simulink model "Misil_Simulink"  (R2021b)
settings: Solver=ode45  StartTime=0.0  StopTime=10  RelTol=1e-3  EnableMultiTasking=on
PreLoadFcn:
  | codigos
undefined symbols (not defined in the file): b_ala, b_est, c, Cd0, CL0, Cl_deltaa, Cl_p, CLalpha, Cm_deltae, Cm_fq, Cm_w, Cn_deltar, Cn_fr, Cn_v, e, g, h, Ix, Ixz, Iy, Iz, L_ala, L_est, Long, m
libraries: aerolibanim x1, aerolibatmos2 x1
settings Model: Creator=usuario  LastModifiedBy=verti
settings SolverCC: AlgebraicLoopSolver=TrustRegion
settings DataIOCC: LimitDataPoints=on  SaveFormat=Array  SignalLoggingSaveFormat=ModelDataLogs  ReturnWorkspaceOutputs=off
settings OptimizationCC: ExpressionDepthLimit=2147483647  LifeSpan=inf
settings DebuggingCC: UnderspecifiedInitializationDetection=Classic  MergeDetectMultiDrivingBlocksExec=none  SolverPrmCheckMsg=warning  FcnCallInpInsideContextMsg=warning  StateNameClashWarn=warning  SFUnexpectedBacktrackingDiag=warning  SFNoUnconditionalDefaultTransitionDiag=warning  SFExecutionAtInitializationDiag=none  SFMachineParentedDataDiag=warning  ArithmeticOperatorsInVariantConditions=warning
settings HardwareCC: ProdBitPerPointer=32  ProdBitPerSizeT=32  ProdBitPerPtrDiffT=32  ProdLargestAtomicFloat=None  ProdIntDivRoundTo=Undefined  ProdEndianess=Unspecified  ProdWordSize=32  ProdHWDeviceType=32-bit Generic
settings ModelReferenceCC: PropagateSignalLabelsOutOfModel=off
settings SFSimCC: SimUseLocalCustomCode=off  CustomCodeUndefinedFunction=UseInterfaceOnly
settings RTWCC: RTWUseLocalCustomCode=off
settings CodeAppCC: StateflowObjectComments=on
settings GRTTargetCC: TargetLangStandard=C89/C90 (ANSI)  CombineOutputUpdateFcns=off  GRTInterface=on
settings ConfigComp: CovMetricSettings=dw  CovSaveCumulativeToWorkspaceVar=on  CovSaveSingleToWorkspaceVar=on  CovExternalEMLEnable=off

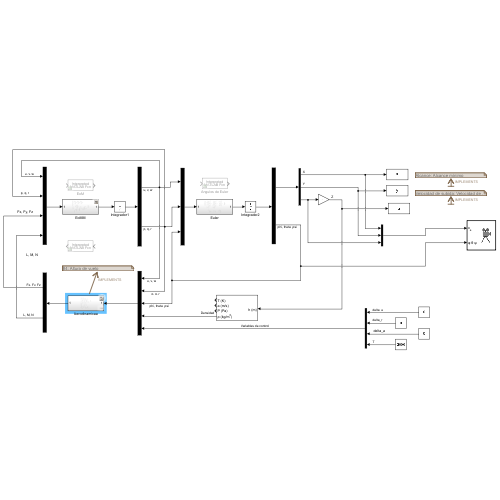
[thumbnail: Simulink's stored preview of the top-level diagram]
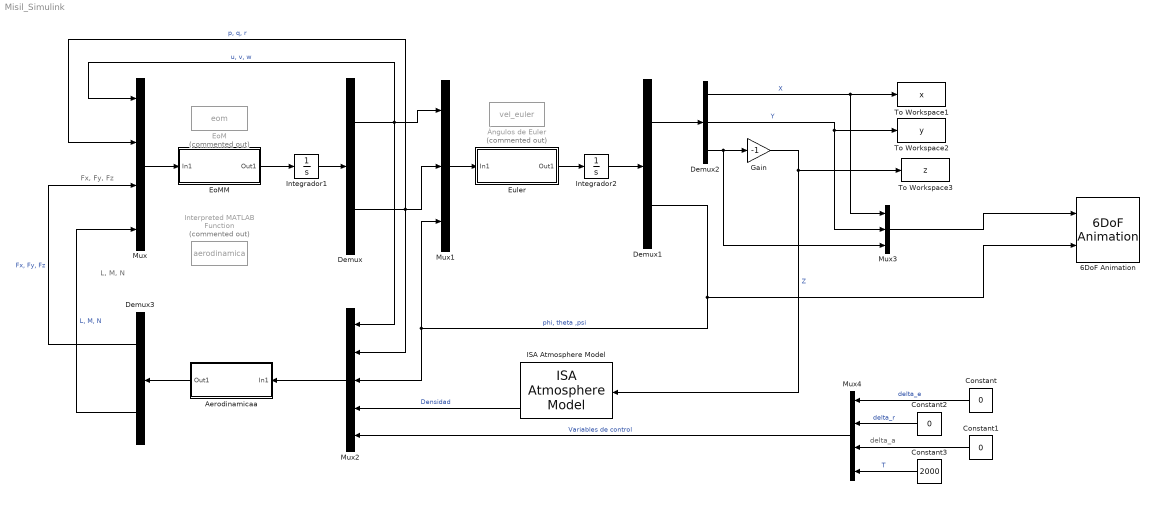
== system Misil_Simulink ==
  note: delta_a
  note: Fx, Fy, Fz
  note: L, M, N
  6DoF Animation : aerolibanim/6DoF Animation  u1=[0 4000 0 4000 0 4000]  u2=0.1  u3=20  u4=[0 0 0]  u5=Fly alongside  u6=[200 200 200]  u7=10  u8=on
  Aerodinamicaa : Subsystem
  Constant : Constant  Value=0
  Constant1 : Constant  Value=0
  Constant2 : Constant  Value=0
  Constant3 : Constant  Value=2000
  Demux : Demux  Outputs=2
  Demux1 : Demux  Outputs=2
  Demux2 : Demux  Outputs=3
  Demux3 : Demux  Outputs=2
  EoM : MATLABFcn  Commented=on  MATLABFcn=eom  OutputDimensions=6
  EoMM : Subsystem
  Euler : Subsystem
  Gain : Gain  Gain=-1
  ISA Atmosphere Model : aerolibatmos2/ISA Atmosphere Model  custom=off  g=9.80665  gamma=1.4  R=287.0531  L=0.0065  h_trop=11000  h_strat=20000  rho0=1.225  P0=101325  T0=288.15  h0=0
  Integrador1 : Integrator  InitialCondition=[0.001,0,0,0,0,0]
  Integrador2 : Integrator  InitialCondition=[0,0,2000,0,pi/4,0]
      settings: DeleteFcn=slcm Cancel;  NameChangeFcn=slcm Rename;
  Interpreted MATLAB Function : MATLABFcn  Commented=on  MATLABFcn=aerodinamica  OutputDimensions=6
  Mux : Mux
  Mux1 : Mux  Inputs=3
  Mux2 : Mux  Inputs=5
  Mux3 : Mux  Inputs=3
  Mux4 : Mux
  To Workspace1 : ToWorkspace  VariableName=x  SampleTime=-1
  To Workspace2 : ToWorkspace  VariableName=y  SampleTime=-1
  To Workspace3 : ToWorkspace  VariableName=z  SampleTime=-1
  Ángulos de Euler : MATLABFcn  Commented=on  MATLABFcn=vel_euler  OutputDimensions=6
  wires:
  Integrador1/1 -> Demux/1
  Mux1/1 -> Euler/1(In1)
  Integrador2/1 -> Demux1/1
  Demux1/1 -> Demux2/1
  Demux/2 -> Mux2/2, Mux/2, Mux1/2  "p, q, r"
  Demux1/2 -> 6DoF Animation/2, Mux2/3, Mux1/3  "phi, theta ,psi"
  Demux2/3 -> Gain/1, Mux3/3
  Gain/1 -> ISA Atmosphere Model/1, To Workspace3/1  "Z"
  Demux2/1 -> Mux3/1, To Workspace1/1  "X"
  Demux2/2 -> Mux3/2, To Workspace2/1  "Y"
  Constant3/1 -> Mux4/4  "T"
  Constant1/1 -> Mux4/3
  Constant2/1 -> Mux4/2  "delta_r"
  Constant/1 -> Mux4/1  "delta_e"
  Demux3/1 -> Mux/3  "Fx, Fy, Fz"
  Demux3/2 -> Mux/4  "L, M, N"
  ISA Atmosphere Model/4 -> Mux2/4  "Densidad"
  Mux4/1 -> Mux2/5  "Variables de control"
  Mux3/1 -> 6DoF Animation/1
  Demux/1 -> Mux2/1, Mux/1, Mux1/1  "u, v, w"
  Mux2/1 -> Aerodinamicaa/1(In1)
  Aerodinamicaa/1(Out1) -> Demux3/1
  Mux/1 -> EoMM/1(In1)
  EoMM/1(Out1) -> Integrador1/1
  Euler/1(Out1) -> Integrador2/1

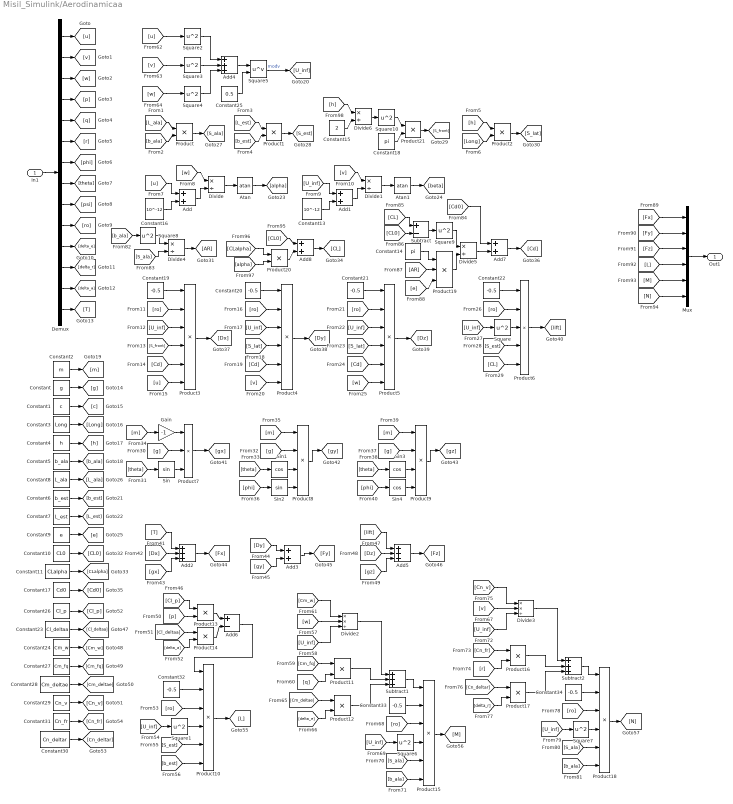
== system Misil_Simulink/Aerodinamicaa ==
  In1 : Inport
  Add{,1,3,7..8} (5 alike) : Sum
  Add2 : Sum  Inputs=+++
  Add4 : Sum  Inputs=+++
  Add5 : Sum  Inputs=+++
  Add6 : Sum  Inputs=+-
  Atan : Trigonometry  Operator=atan
  Atan1 : Trigonometry  Operator=atan
  Constant : Constant  Value=g
  Constant1 : Constant  Value=c
  Constant10 : Constant  Value=CL0
  Constant11 : Constant  Value=CLalpha
  Constant13 : Constant  Value=10^-12
  Constant14 : Constant  Value=pi
  Constant15 : Constant  Value=2
  Constant16 : Constant  Value=10^-12
  Constant17 : Constant  Value=Cd0
  Constant18 : Constant  Value=pi
  Constant{19..22,32..34} (7 alike) : Constant  Value=-0.5
  Constant2 : Constant  Value=m
  Constant23 : Constant  Value=Cl_deltaa
  Constant24 : Constant  Value=Cm_w
  Constant25 : Constant  Value=0.5
  Constant26 : Constant  Value=Cl_p
  Constant27 : Constant  Value=Cm_fq
  Constant28 : Constant  Value=Cm_deltae
  Constant29 : Constant  Value=Cn_v
  Constant3 : Constant  Value=Long
  Constant30 : Constant  Value=Cn_deltar
  Constant31 : Constant  Value=Cn_fr
  Constant4 : Constant  Value=h
  Constant5 : Constant  Value=b_ala
  Constant6 : Constant  Value=b_est
  Constant7 : Constant  Value=L_est
  Constant8 : Constant  Value=L_ala
  Constant9 : Constant  Value=e
  Demux : Demux  Outputs=14
  Divide{,1,4..6} (5 alike) : Product  Inputs=*/
  Divide2 : Product  Inputs=**/
  Divide3 : Product  Inputs=**/
  Gain : Gain  Gain=-1
  Mux : Mux  Inputs=6
  Product{,1..2,11..14,16..17,20..21} (11 alike) : Product
  Product{3..5,10,15,18} (6 alike) : Product  Inputs=6
  Product19 : Product  Inputs=3
  Product6 : Product  Inputs=5
  Product7 : Product  Inputs=3
  Product8 : Product  Inputs=4
  Product9 : Product  Inputs=4
  Sin : Trigonometry
  Sin1 : Trigonometry  Operator=cos
  Sin2 : Trigonometry
  Sin3 : Trigonometry  Operator=cos
  Sin4 : Trigonometry  Operator=cos
  Square{,1..4,6..10} (10 alike) : Math  Operator=square  SaturateOnIntegerOverflow=on
  Square5 : Math  Operator=pow  SaturateOnIntegerOverflow=on
  Subtract : Sum  Inputs=+-
  Subtract1 : Sum  Inputs=+++
  Subtract2 : Sum  Inputs=+++
  Out1 : Outport
  wires:
  In1/1 -> Demux/1
  Mux/1 -> Out1/1
  Demux/1 -> [u]
  Demux/2 -> [v]
  Demux/6 -> [r]
  Demux/5 -> [q]
  Demux/4 -> [p]
  Demux/3 -> [w]
  Demux/7 -> [phi]
  Demux/14 -> [T]
  Demux/13 -> [delta_a]
  Demux/12 -> [delta_r]
  Demux/11 -> [delta_e]
  Demux/10 -> [ro]
  Demux/9 -> [psi]
  Demux/8 -> [theta]
  Constant3/1 -> [Long]
  Constant2/1 -> [m]
  Constant/1 -> [g]
  Constant4/1 -> [h]
  Constant5/1 -> [b_ala]
  Constant1/1 -> [c]
  Add4/1 -> Square5/1
  Square5/1 -> [U_inf]  "modv"
  Constant25/1 -> Square5/2
  Square3/1 -> Add4/2
  [w] -> Square4/1
  [v] -> Square3/1
  Square4/1 -> Add4/3
  Square2/1 -> Add4/1
  [u] -> Square2/1
  Constant7/1 -> [L_est]
  Constant11/1 -> [CLalpha]
  Constant10/1 -> [CL0]
  Constant6/1 -> [b_est]
  Constant9/1 -> [e]
  [L_ala] -> Product/1
  [b_ala] -> Product/2
  Product/1 -> [S_ala]
  Product1/1 -> [S_est]
  [b_est] -> Product1/2
  [L_est] -> Product1/1
  [h] -> Product2/1
  Product2/1 -> [S_lat]
  [Long] -> Product2/2
  [u] -> Add/1
  Divide/1 -> Atan/1
  Add/1 -> Divide/2
  Atan/1 -> [alpha]
  [w] -> Divide/1
  Constant16/1 -> Add/2
  Constant13/1 -> Add1/2
  [v] -> Divide1/1
  Atan1/1 -> [beta]
  Add1/1 -> Divide1/2
  Divide1/1 -> Atan1/1
  [U_inf] -> Add1/1
  Divide4/1 -> [AR]
  Constant17/1 -> [Cd0]
  [U_inf] -> Product3/3
  [ro] -> Product3/2
  [Cd] -> Product3/5
  Constant19/1 -> Product3/1
  Product3/1 -> [Dx]
  [u] -> Product3/6
  [S_front] -> Product3/4
  [S_lat] -> Product4/4
  [v] -> Product4/6
  Product4/1 -> [Dy]
  Constant20/1 -> Product4/1
  [Cd] -> Product4/5
  [ro] -> Product4/2
  [U_inf] -> Product4/3
  [U_inf] -> Product5/3
  [ro] -> Product5/2
  [Cd] -> Product5/5
  Constant21/1 -> Product5/1
  Product5/1 -> [Dz]
  [w] -> Product5/6
  [S_lat] -> Product5/4
  [S_est] -> Product6/4
  Product6/1 -> [lift]
  Constant22/1 -> Product6/1
  [CL] -> Product6/5
  [ro] -> Product6/2
  [U_inf] -> Square/1
  Square/1 -> Product6/3
  Gain/1 -> Product7/1
  [g] -> Product7/2
  [theta] -> Sin/1
  Sin/1 -> Product7/3
  Product7/1 -> [gx]
  Product8/1 -> [gy]
  Sin1/1 -> Product8/3
  [theta] -> Sin1/1
  [g] -> Product8/2
  [m] -> Product8/1
  [m] -> Gain/1
  [phi] -> Sin2/1
  Sin2/1 -> Product8/4
  Sin4/1 -> Product9/4
  [phi] -> Sin4/1
  [m] -> Product9/1
  [g] -> Product9/2
  [theta] -> Sin3/1
  Sin3/1 -> Product9/3
  Product9/1 -> [gz]
  [T] -> Add2/1
  [Dx] -> Add2/2
  [gx] -> Add2/3
  Add2/1 -> [Fx]
  [gy] -> Add3/2
  Add3/1 -> [Fy]
  [Dy] -> Add3/1
  [lift] -> Add5/1
  Add5/1 -> [Fz]
  [gz] -> Add5/3
  [Dz] -> Add5/2
  Constant30/1 -> [Cn_deltar]
  Constant24/1 -> [Cm_w]
  Constant29/1 -> [Cn_v]
  Constant28/1 -> [Cm_deltae]
  Constant23/1 -> [Cl_deltaa]
  Constant26/1 -> [Cl_p]
  Constant27/1 -> [Cm_fq]
  Constant31/1 -> [Cn_fr]
  [Cl_p] -> Product13/1
  Product14/1 -> Add6/2
  [Cl_deltaa] -> Product14/1
  [p] -> Product13/2
  [delta_a] -> Product14/2
  [ro] -> Product10/3
  Square1/1 -> Product10/4
  [b_est] -> Product10/6
  Constant32/1 -> Product10/2
  Add6/1 -> Product10/1
  [U_inf] -> Square1/1
  Product10/1 -> [L]
  Product13/1 -> Add6/1
  [S_est] -> Product10/5
  Product15/1 -> [M]
  [Cm_fq] -> Product11/1
  [Cm_w] -> Divide2/1
  [S_ala] -> Product15/5
  [U_inf] -> Square6/1
  Divide2/1 -> Subtract1/1
  [w] -> Divide2/2
  [b_ala] -> Product15/6
  [ro] -> Product15/3
  Subtract1/1 -> Product15/1
  [U_inf] -> Divide2/3
  Constant33/1 -> Product15/2
  Product11/1 -> Subtract1/2
  [q] -> Product11/2
  Square6/1 -> Product15/4
  [delta_e] -> Product12/2
  [Cm_deltae] -> Product12/1
  Product12/1 -> Subtract1/3
  Product17/1 -> Subtract2/3
  [Cn_deltar] -> Product17/1
  [delta_r] -> Product17/2
  Square7/1 -> Product18/4
  [r] -> Product16/2
  Product16/1 -> Subtract2/2
  Constant34/1 -> Product18/2
  [U_inf] -> Divide3/3
  Subtract2/1 -> Product18/1
  [ro] -> Product18/3
  [b_ala] -> Product18/6
  [v] -> Divide3/2
  Divide3/1 -> Subtract2/1
  [U_inf] -> Square7/1
  [S_ala] -> Product18/5
  [Cn_v] -> Divide3/1
  [Cn_fr] -> Product16/1
  Product18/1 -> [N]
  [b_ala] -> Square8/1
  [S_ala] -> Divide4/2
  Square8/1 -> Divide4/1
  Add7/1 -> [Cd]
  [Cd0] -> Add7/1
  [CL0] -> Subtract/2
  [CL] -> Subtract/1
  Subtract/1 -> Square9/1
  Square9/1 -> Divide5/1
  Product19/1 -> Divide5/2
  Constant14/1 -> Product19/1
  [AR] -> Product19/2
  [e] -> Product19/3
  Divide5/1 -> Add7/2
  [Fx] -> Mux/1
  [Fy] -> Mux/2
  [Fz] -> Mux/3
  [L] -> Mux/4
  [M] -> Mux/5
  [N] -> Mux/6
  Add8/1 -> [CL]
  Product20/1 -> Add8/2
  [CL0] -> Add8/1
  [alpha] -> Product20/2
  [CLalpha] -> Product20/1
  [h] -> Divide6/1
  Constant15/1 -> Divide6/2
  Product21/1 -> [S_front]
  Divide6/1 -> Square10/1
  Constant18/1 -> Product21/2
  Square10/1 -> Product21/1
  Constant8/1 -> [L_ala]

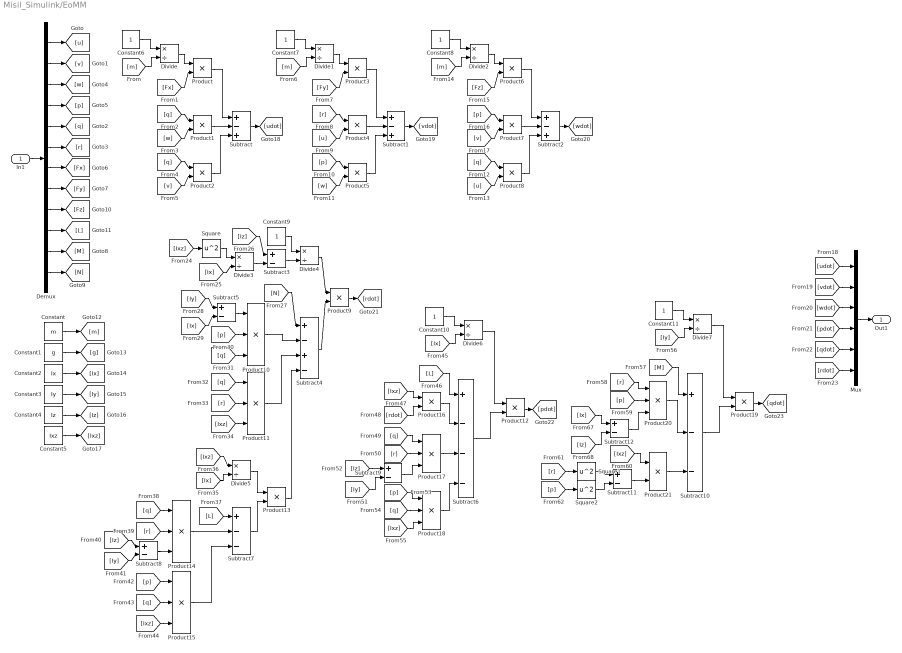
== system Misil_Simulink/EoMM ==
  In1 : Inport
  Constant : Constant  Value=m
  Constant1 : Constant  Value=g
  Constant{6..11} (6 alike) : Constant
  Constant2 : Constant  Value=Ix
  Constant3 : Constant  Value=Iy
  Constant4 : Constant  Value=Iz
  Constant5 : Constant  Value=Ixz
  Demux : Demux  Outputs=12
  Divide{,1..7} (8 alike) : Product  Inputs=*/
  Mux : Mux  Inputs=6
  Product{,1..9,12..13,16,19,21} (15 alike) : Product
  Product{10..11,14..15,17..18,20} (7 alike) : Product  Inputs=3
  Square : Math  Operator=square  SaturateOnIntegerOverflow=on
  Square1 : Math  Operator=square  SaturateOnIntegerOverflow=on
  Square2 : Math  Operator=square  SaturateOnIntegerOverflow=on
  Subtract : Sum  Inputs=+-+
  Subtract1 : Sum  Inputs=+-+
  Subtract10 : Sum  Inputs=+--
  Subtract{3,5,8..9,11..12} (6 alike) : Sum  Inputs=+-
  Subtract2 : Sum  Inputs=+-+
  Subtract4 : Sum  Inputs=+-+-
  Subtract6 : Sum  Inputs=+---
  Subtract7 : Sum  Inputs=+--
  Out1 : Outport
  wires:
  In1/1 -> Demux/1
  Demux/3 -> [w]
  Demux/1 -> [u]
  Demux/2 -> [v]
  Demux/4 -> [p]
  Demux/5 -> [q]
  Demux/6 -> [r]
  Demux/7 -> [Fx]
  Demux/12 -> [N]
  Demux/11 -> [M]
  Demux/10 -> [L]
  Demux/9 -> [Fz]
  Demux/8 -> [Fy]
  Constant/1 -> [m]
  Constant1/1 -> [g]
  Constant3/1 -> [Iy]
  Constant2/1 -> [Ix]
  Constant5/1 -> [Ixz]
  Constant4/1 -> [Iz]
  Constant6/1 -> Divide/1
  [m] -> Divide/2
  [Fx] -> Product/2
  Divide/1 -> Product/1
  [q] -> Product1/1
  [w] -> Product1/2
  [q] -> Product2/1
  [v] -> Product2/2
  Product2/1 -> Subtract/3
  Product/1 -> Subtract/1
  Product1/1 -> Subtract/2
  Subtract/1 -> [udot]
  Subtract1/1 -> [vdot]
  Product4/1 -> Subtract1/2
  Product3/1 -> Subtract1/1
  Product5/1 -> Subtract1/3
  [w] -> Product5/2
  [p] -> Product5/1
  [u] -> Product4/2
  [r] -> Product4/1
  Divide1/1 -> Product3/1
  [Fy] -> Product3/2
  [m] -> Divide1/2
  Constant7/1 -> Divide1/1
  Constant8/1 -> Divide2/1
  [m] -> Divide2/2
  [Fz] -> Product6/2
  Divide2/1 -> Product6/1
  [p] -> Product7/1
  [v] -> Product7/2
  [q] -> Product8/1
  [u] -> Product8/2
  Product8/1 -> Subtract2/3
  Product6/1 -> Subtract2/1
  Product7/1 -> Subtract2/2
  Subtract2/1 -> [wdot]
  [rdot] -> Mux/6
  Mux/1 -> Out1/1
  [udot] -> Mux/1
  [vdot] -> Mux/2
  [wdot] -> Mux/3
  [pdot] -> Mux/4
  [qdot] -> Mux/5
  [Ixz] -> Square/1
  Square/1 -> Divide3/1
  [Ix] -> Divide3/2
  [Iz] -> Subtract3/1
  Divide3/1 -> Subtract3/2
  Subtract3/1 -> Divide4/2
  Constant9/1 -> Divide4/1
  Divide4/1 -> Product9/1
  Subtract4/1 -> Product9/2
  [N] -> Subtract4/1
  [Iy] -> Subtract5/1
  [Ix] -> Subtract5/2
  Subtract5/1 -> Product10/1
  Product10/1 -> Subtract4/2
  [p] -> Product10/2
  [q] -> Product10/3
  [Ixz] -> Product11/3
  [r] -> Product11/2
  Product11/1 -> Subtract4/3
  [q] -> Product11/1
  [Ix] -> Divide5/2
  [Ixz] -> Divide5/1
  Product13/1 -> Subtract4/4
  Divide5/1 -> Product13/1
  Subtract7/1 -> Product13/2
  [L] -> Subtract7/1
  Product14/1 -> Subtract7/2
  Subtract8/1 -> Product14/3
  [q] -> Product14/1
  [r] -> Product14/2
  [Iz] -> Subtract8/1
  [Iy] -> Subtract8/2
  [q] -> Product15/2
  [p] -> Product15/1
  Product15/1 -> Subtract7/3
  [Ixz] -> Product15/3
  Product9/1 -> [rdot]
  Product12/1 -> [pdot]
  [Ix] -> Divide6/2
  Constant10/1 -> Divide6/1
  Divide6/1 -> Product12/1
  Subtract6/1 -> Product12/2
  [L] -> Subtract6/1
  [Ixz] -> Product16/1
  [rdot] -> Product16/2
  Product16/1 -> Subtract6/2
  Product17/1 -> Subtract6/3
  [q] -> Product17/1
  [r] -> Product17/2
  Subtract9/1 -> Product17/3
  [Iz] -> Subtract9/1
  [Iy] -> Subtract9/2
  [q] -> Product18/2
  [p] -> Product18/1
  [Ixz] -> Product18/3
  Product18/1 -> Subtract6/4
  [Ixz] -> Product21/1
  Product21/1 -> Subtract10/3
  Product20/1 -> Subtract10/2
  [M] -> Subtract10/1
  Subtract10/1 -> Product19/2
  Divide7/1 -> Product19/1
  Constant11/1 -> Divide7/1
  [Iy] -> Divide7/2
  Product19/1 -> [qdot]
  [r] -> Product20/1
  [p] -> Product20/2
  Subtract12/1 -> Product20/3
  [Ix] -> Subtract12/1
  [Iz] -> Subtract12/2
  Subtract11/1 -> Product21/2
  [r] -> Square1/1
  [p] -> Square2/1
  Square2/1 -> Subtract11/2
  Square1/1 -> Subtract11/1

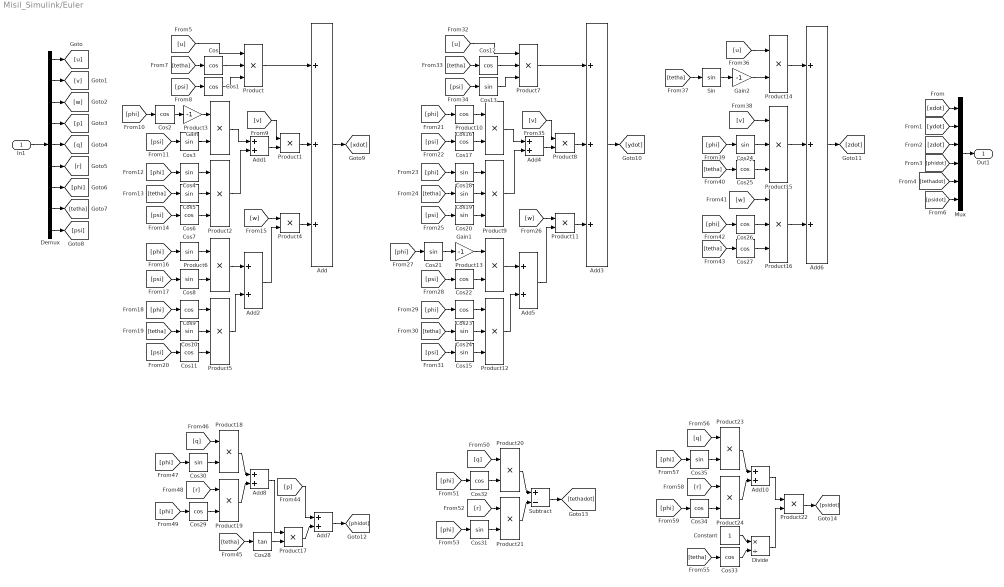
== system Misil_Simulink/Euler ==
  In1 : Inport
  Add : Sum  Inputs=+++
  Add{1..2,4..5,7..8,10} (7 alike) : Sum
  Add3 : Sum  Inputs=+++
  Add6 : Sum  Inputs=+++
  Constant : Constant
  Cos{,1..2,6,9,11..12,16..17,22..23,25..27,29,32..34} (18 alike) : Trigonometry  Operator=cos
  Cos{3..5,7..8,10,13..15,18..21,24,30..31,35} (17 alike) : Trigonometry
  Cos28 : Trigonometry  Operator=tan
  Demux : Demux  Outputs=9
  Divide : Product  Inputs=*/
  Gain : Gain  Gain=-1
  Gain1 : Gain  Gain=-1
  Gain2 : Gain  Gain=-1
  Mux : Mux  Inputs=6
  Product{,2,5,7,9,12,15..16} (8 alike) : Product  Inputs=3
  Product{1,3..4,6,8,10..11,13..14,17..24} (17 alike) : Product
  Sin : Trigonometry
  Subtract : Sum  Inputs=+-
  Out1 : Outport
  wires:
  In1/1 -> Demux/1
  Demux/1 -> [u]
  Demux/2 -> [v]
  Demux/3 -> [w]
  Demux/4 -> [p]
  Demux/5 -> [q]
  Demux/6 -> [r]
  Demux/7 -> [phi]
  Demux/8 -> [tetha]
  Demux/9 -> [psi]
  Mux/1 -> Out1/1
  [xdot] -> Mux/1
  [ydot] -> Mux/2
  [tethadot] -> Mux/5
  [psidot] -> Mux/6
  [phidot] -> Mux/4
  [zdot] -> Mux/3
  Add/1 -> [xdot]
  [psi] -> Cos1/1
  [tetha] -> Cos/1
  Cos1/1 -> Product/3
  Cos/1 -> Product/2
  [u] -> Product/1
  Product/1 -> Add/1
  Product1/1 -> Add/2
  [v] -> Product1/1
  Add1/1 -> Product1/2
  Product2/1 -> Add1/2
  Product3/1 -> Add1/1
  [phi] -> Cos2/1
  Cos2/1 -> Gain/1
  Gain/1 -> Product3/1
  Cos3/1 -> Product3/2
  [psi] -> Cos3/1
  [phi] -> Cos4/1
  [tetha] -> Cos5/1
  [psi] -> Cos6/1
  Cos5/1 -> Product2/2
  Cos4/1 -> Product2/1
  Cos6/1 -> Product2/3
  Add2/1 -> Product4/2
  [w] -> Product4/1
  Product4/1 -> Add/3
  Cos11/1 -> Product5/3
  Cos9/1 -> Product5/1
  Cos10/1 -> Product5/2
  [psi] -> Cos11/1
  [tetha] -> Cos10/1
  [phi] -> Cos9/1
  [psi] -> Cos8/1
  Cos8/1 -> Product6/2
  Cos7/1 -> Product6/1
  [phi] -> Cos7/1
  Product6/1 -> Add2/1
  Product5/1 -> Add2/2
  Product12/1 -> Add5/2
  Product13/1 -> Add5/1
  [phi] -> Cos21/1
  Cos21/1 -> Gain1/1
  Cos22/1 -> Product13/2
  [psi] -> Cos22/1
  [phi] -> Cos23/1
  [tetha] -> Cos14/1
  [psi] -> Cos15/1
  Cos14/1 -> Product12/2
  Cos23/1 -> Product12/1
  Cos15/1 -> Product12/3
  Product11/1 -> Add3/3
  [w] -> Product11/1
  Add5/1 -> Product11/2
  Cos20/1 -> Product9/3
  Cos18/1 -> Product9/1
  Cos19/1 -> Product9/2
  [psi] -> Cos20/1
  [tetha] -> Cos19/1
  [phi] -> Cos18/1
  [psi] -> Cos17/1
  Cos17/1 -> Product10/2
  Cos16/1 -> Product10/1
  [phi] -> Cos16/1
  Product10/1 -> Add4/1
  Product9/1 -> Add4/2
  Add4/1 -> Product8/2
  [v] -> Product8/1
  Product8/1 -> Add3/2
  Product7/1 -> Add3/1
  [u] -> Product7/1
  Cos12/1 -> Product7/2
  Cos13/1 -> Product7/3
  [tetha] -> Cos12/1
  [psi] -> Cos13/1
  Add3/1 -> [ydot]
  Gain1/1 -> Product13/1
  Add6/1 -> [zdot]
  Product14/1 -> Add6/1
  [u] -> Product14/1
  [tetha] -> Sin/1
  Sin/1 -> Gain2/1
  Gain2/1 -> Product14/2
  Product15/1 -> Add6/2
  [v] -> Product15/1
  [phi] -> Cos24/1
  [tetha] -> Cos25/1
  Cos25/1 -> Product15/3
  Cos24/1 -> Product15/2
  Cos26/1 -> Product16/2
  Cos27/1 -> Product16/3
  [tetha] -> Cos27/1
  [phi] -> Cos26/1
  [w] -> Product16/1
  Product16/1 -> Add6/3
  Add7/1 -> [phidot]
  [p] -> Add7/1
  Product17/1 -> Add7/2
  Add8/1 -> Product17/1
  [tetha] -> Cos28/1
  Cos28/1 -> Product17/2
  [q] -> Product18/1
  Cos30/1 -> Product18/2
  [phi] -> Cos30/1
  Product18/1 -> Add8/1
  [phi] -> Cos29/1
  Cos29/1 -> Product19/2
  [r] -> Product19/1
  Product19/1 -> Add8/2
  Product21/1 -> Subtract/2
  [r] -> Product21/1
  Cos31/1 -> Product21/2
  [phi] -> Cos31/1
  Product20/1 -> Subtract/1
  [phi] -> Cos32/1
  Cos32/1 -> Product20/2
  [q] -> Product20/1
  Subtract/1 -> [tethadot]
  Product24/1 -> Add10/2
  [r] -> Product24/1
  Cos34/1 -> Product24/2
  [phi] -> Cos34/1
  Product23/1 -> Add10/1
  [phi] -> Cos35/1
  Cos35/1 -> Product23/2
  [q] -> Product23/1
  [tetha] -> Cos33/1
  Add10/1 -> Product22/1
  Product22/1 -> [psidot]
  Constant/1 -> Divide/1
  Cos33/1 -> Divide/2
  Divide/1 -> Product22/2
